simulink subsystem "Day1_Scenario_3_4"  (R2024a)
settings: Solver=VariableStepAuto  StartTime=0.0  StopTime=10.0  RelTol=1e-3
libraries: CarMaker4SL x3
settings Model: Creator=junhyung.cha  LastModifiedBy=User

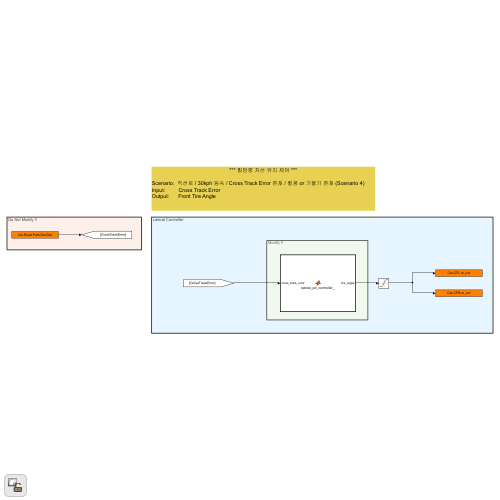
[thumbnail: Simulink's stored preview of the top-level diagram]
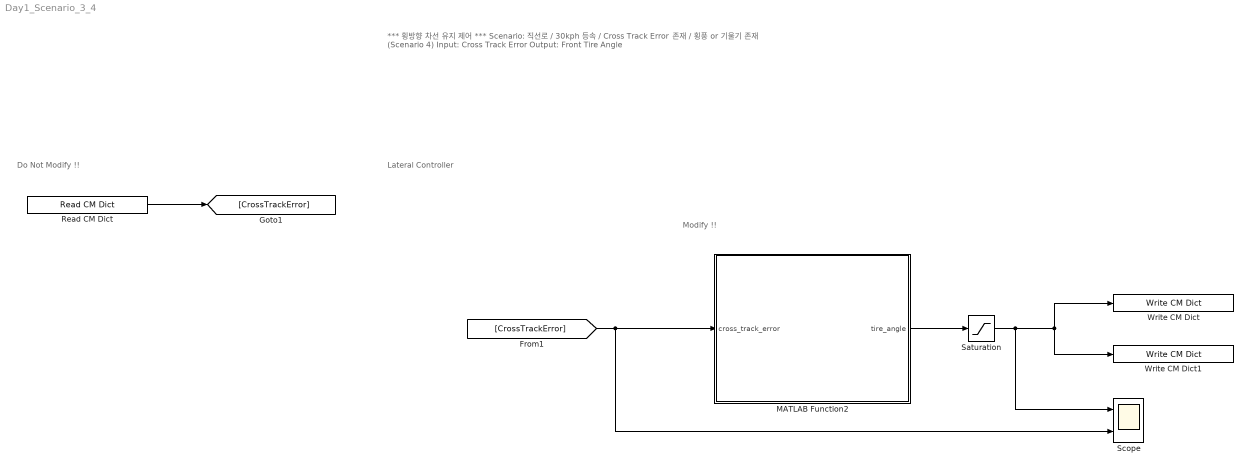
== system Day1_Scenario_3_4 ==
  note: Do Not Modify !!
  note: Modify !!
  note: Lateral Controller
  note: *** 횡방향 차선 유지 제어 ***
      |
      | Scenario: 직선로 / 30kph 등속 / Cross Track Error 존재 / 횡풍 or 기울기 존재 (Scenario 4)
      | Input: Cross Track Error
      | Output: Front Tire Angle
  MATLAB Function2 : MATLAB Function  TreatAsAtomicUnit=on
  Read CM Dict : CarMaker4SL/Read CM Dict  xname=Car.Road.Path.DevDist  xsync=off  xstime=Inherited
  Saturation : Saturate  UpperLimit=2  LowerLimit=-2
  Scope : Scope  NumInputPorts=2
  Write CM Dict : CarMaker4SL/Write CM Dict  xname=Car.CFL.rz_ext  xsync=off
  Write CM Dict1 : CarMaker4SL/Write CM Dict  xname=Car.CFR.rz_ext  xsync=off
  wires:
  Read CM Dict/1 -> [CrossTrackError]
  MATLAB Function2/1(tire_angle) -> Saturation/1
  [CrossTrackError] -> MATLAB Function2/1(cross_track_error), Scope/2
  Saturation/1 -> Write CM Dict/1, Write CM Dict1/1, Scope/1

== matlab function Day1_Scenario_3_4/MATLAB Function2 ==
  settings: updateMethod=DISCRETE  sampleTime=0.05
  data: cross_track_error input; tire_angle output
function tire_angle = lateral_pd_controller_(cross_track_error)
    tire_angle = 0;
    % lateral_pd_controller_  단순 PD 횡방향 제어기
%
%   입력:
%     cross_track_error  – 차선 중앙에서 벗어난 거리 (m)
%   출력:
%     tire_angle         – 조향각 명령치 (rad)

  %#codegen
  persistent Kp Kd dt prev_cte
  if isempty(Kp)
    % — Python 예제와 동일한 이득 & 샘플타임 사용 —
    Kp       = -0.24;    % P 이득
    Kd       = 0.04;    % D 이득
    dt       = 0.1;    % 샘플 간격 [s]
    prev_cte = 0.0;    % 이전 CTE 초기화
  end

  % 1) 현재 오차
  cte = cross_track_error;

  % 2) 오차 변화율 (미분항)
  dcte = (cte - prev_cte) / dt;

  % 3) PD 제어 법칙
  tire_angle = Kp * cte + Kd * dcte;

  % 4) 상태 업데이트
  prev_cte = cte;
end
